simulink model "main_2022b"  (R2022b)
settings: Solver=ode4  StartTime=0.0  StopTime=0.1  FixedStep=deltat  RelTol=1e-3
model workspace (MAT data in the model file):
  Dutyfactor = Simulink.Parameter
  Dutyfactor.Value = 0.25
  Dutyfactor.DataType = 'double'
  Dutyfactor.Complexity = 'real'
  Dutyfactor.Dimensions = [1 1]
  LenghtOfBot = Simulink.Parameter
  LenghtOfBot.Value = 0.5
  LenghtOfBot.DataType = 'double'
  LenghtOfBot.Complexity = 'real'
  LenghtOfBot.Dimensions = [1 1]
  MomentOfInertia = Simulink.Parameter
  MomentOfInertia.Value = [0.41  0  0; 0  2.1  0; 0  0  2.1]
  MomentOfInertia.DataType = 'double'
  MomentOfInertia.Complexity = 'real'
  MomentOfInertia.Dimensions = [3 3]
  RelativePhase = Simulink.Parameter
  RelativePhase.Value = [0; 0.5; 0.75; 0.25]
  RelativePhase.DataType = 'double'
  RelativePhase.Complexity = 'real'
  RelativePhase.Dimensions = [4 1]
  WidthOfBot = Simulink.Parameter
  WidthOfBot.Value = 0.3
  WidthOfBot.DataType = 'double'
  WidthOfBot.Complexity = 'real'
  WidthOfBot.Dimensions = [1 1]
  cycleTime = Simulink.Parameter
  cycleTime.Value = 1
  cycleTime.DataType = 'double'
  cycleTime.Complexity = 'real'
  cycleTime.Dimensions = [1 1]
  deltat = Simulink.Parameter
  deltat.Value = 0.05
  deltat.DataType = 'double'
  deltat.Complexity = 'real'
  deltat.Dimensions = [1 1]
  gravity = Simulink.Parameter
  gravity.Value = [0; 0; -9.8]
  gravity.DataType = 'double'
  gravity.Complexity = 'real'
  gravity.Dimensions = [3 1]
  mass = Simulink.Parameter
  mass.Value = 45
  mass.DataType = 'double'
  mass.Complexity = 'real'
  mass.Dimensions = [1 1]
  nominal_height = Simulink.Parameter
  nominal_height.Value = 0.2
  nominal_height.DataType = 'double'
  nominal_height.Complexity = 'real'
  nominal_height.Dimensions = [1 1]
  number_of_timeStepsMPC = Simulink.Parameter
  number_of_timeStepsMPC.Value = 1
  number_of_timeStepsMPC.DataType = 'int8'
  number_of_timeStepsMPC.Complexity = 'real'
  number_of_timeStepsMPC.Dimensions = [1 1]
settings Model: Creator=user  LastModifiedBy=user
settings OptimizationCC: ReuseModelBlockBuffer=on

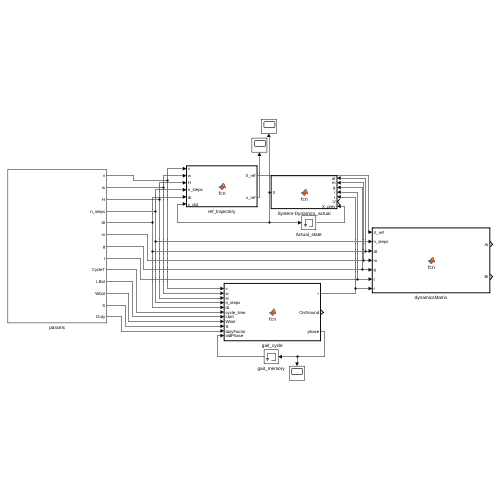
[thumbnail: Simulink's stored preview of the top-level diagram]
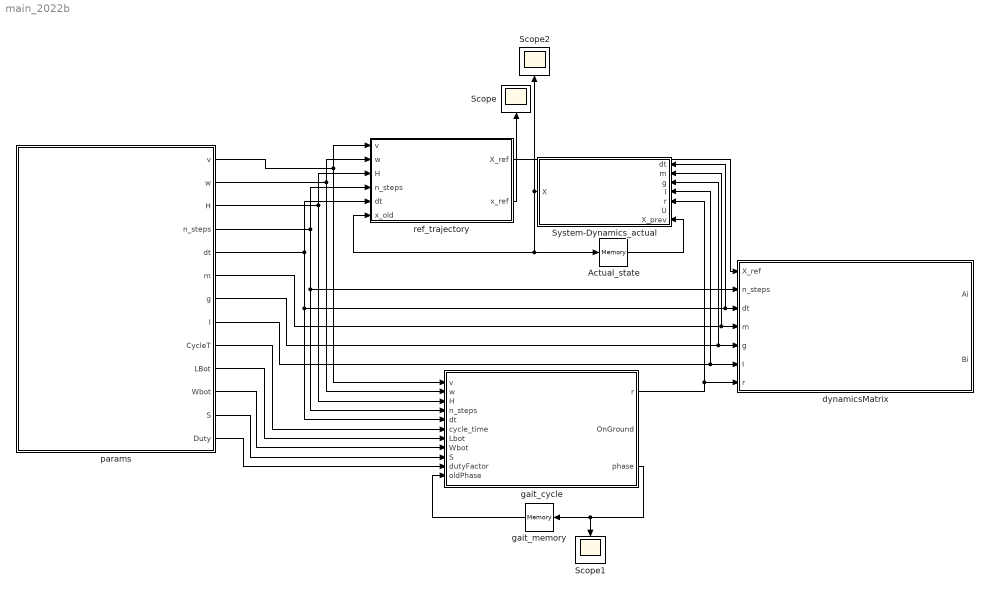
== system main_2022b ==
  Actual_state : Memory
  Scope : Scope
  Scope1 : Scope
  Scope2 : Scope
  System-Dynamics_actual : MATLAB Function  TreatAsAtomicUnit=on
  dynamicsMatrix : MATLAB Function  TreatAsAtomicUnit=on
  gait_cycle : MATLAB Function  TreatAsAtomicUnit=on
  gait_memory : Memory
  params : Subsystem
  ref_trajectory : MATLAB Function  TreatAsAtomicUnit=on
  wires:
  params/1(v) -> ref_trajectory/1(v), gait_cycle/1(v)
  params/2(w) -> gait_cycle/2(w), ref_trajectory/2(w)
  params/3(H) -> gait_cycle/3(H), ref_trajectory/3(H)
  params/4(n_steps) -> gait_cycle/4(n_steps), dynamicsMatrix/2(n_steps), ref_trajectory/4(n_steps)
  ref_trajectory/2(x_ref) -> Scope/1
  params/5(dt) -> gait_cycle/5(dt), dynamicsMatrix/3(dt), System-Dynamics_actual/1(dt), ref_trajectory/5(dt)
  params/9(CycleT) -> gait_cycle/6(cycle_time)
  params/10(LBot) -> gait_cycle/7(Lbot)
  params/11(Wbot) -> gait_cycle/8(Wbot)
  gait_memory/1 -> gait_cycle/11(oldPhase)
  ref_trajectory/1(X_ref) -> dynamicsMatrix/1(X_ref)
  params/6(m) -> dynamicsMatrix/4(m), System-Dynamics_actual/2(m)
  params/7(g) -> dynamicsMatrix/5(g), System-Dynamics_actual/3(g)
  gait_cycle/1(r) -> dynamicsMatrix/7(r), System-Dynamics_actual/5(r)
  params/12(S) -> gait_cycle/9(S)
  params/13(Duty) -> gait_cycle/10(dutyFactor)
  params/8(I) -> dynamicsMatrix/6(I), System-Dynamics_actual/4(I)
  System-Dynamics_actual/1(X) -> ref_trajectory/6(x_old), Actual_state/1, Scope2/1
  Actual_state/1 -> System-Dynamics_actual/7(X_prev)
  gait_cycle/3(phase) -> gait_memory/1, Scope1/1

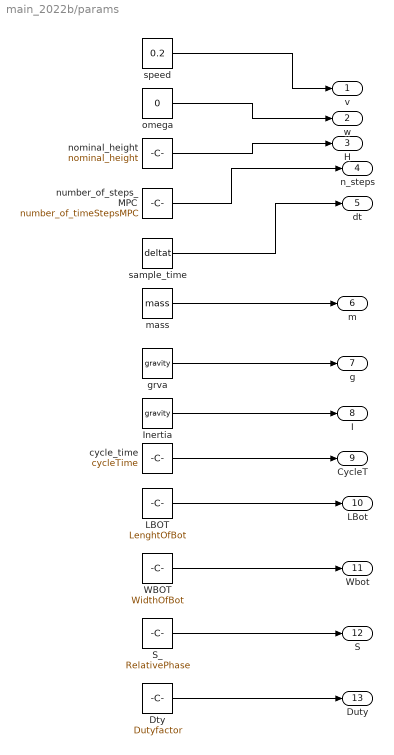
== system main_2022b/params ==
  Dty : Constant  Value=Dutyfactor
  Inertia : Constant  Value=gravity
  LBOT : Constant  Value=LenghtOfBot
  S_ : Constant  Value=RelativePhase
  WBOT : Constant  Value=WidthOfBot
  cycle_time : Constant  Value=cycleTime
  grva : Constant  Value=gravity
  mass : Constant  Value=mass
  nominal_height : Constant  Value=nominal_height
  number_of_steps_MPC : Constant  Value=number_of_timeStepsMPC
  omega : Constant  Value=0
  sample_time : Constant  Value=deltat
  speed : Constant  Value=0.2
  v : Outport
  w : Outport  Port=2
  H : Outport  Port=3
  n_steps : Outport  Port=4
  dt : Outport  Port=5
  m : Outport  Port=6
  g : Outport  Port=7
  I : Outport  Port=8
  CycleT : Outport  Port=9
  LBot : Outport  Port=10
  Wbot : Outport  Port=11
  S : Outport  Port=12
  Duty : Outport  Port=13
  wires:
  number_of_steps_MPC/1 -> n_steps/1
  omega/1 -> w/1
  nominal_height/1 -> H/1
  speed/1 -> v/1
  sample_time/1 -> dt/1
  cycle_time/1 -> CycleT/1
  LBOT/1 -> LBot/1
  WBOT/1 -> Wbot/1
  mass/1 -> m/1
  grva/1 -> g/1
  Dty/1 -> Duty/1
  S_/1 -> S/1
  Inertia/1 -> I/1

== matlab function main_2022b/gait_cycle ==
  data: v input; w input; H input; n_steps input; r output size=[3,4,500]; OnGround output size=[4,500]; dt input; cycle_time input; Lbot input; Wbot input; S input; dutyFactor input; oldPhase input; phase output double size=1
function [r,OnGround,phase] = fcn(v,w,H,n_steps,dt,cycle_time,Lbot,Wbot,S,dutyFactor,oldPhase)
    vr=(2*v+w*Wbot)/2;
    vl=(2*v-w*Wbot)/2;
    LstanceR=cycle_time*(1-dutyFactor)*vl;
    LstanceL=cycle_time*(1-dutyFactor)*vr;
    OnGround=zeros(4,n_steps);
    r=zeros(3,4,n_steps);
    phase=oldPhase;
    for k=1:n_steps
        phase=mod(phase+dt/cycle_time,1);
        for i=1:4           
            phase_leg=mod(phase+S(i),1);
            if(phase_leg>dutyFactor)
                OnGround(i,k)=1;
                if(i==1 || i==3)                 
                    r(:,i,k)=[LstanceL*(phase_leg/dutyFactor -0.5);0;0];             
                else
                    r(:,i,k)=[LstanceR*(phase_leg/dutyFactor -0.5);0;0];
                end                
            else
                r(:,i,k)=[0;0;H*0.25];
            end
        end
        r(:,:,k)=r(:,:,k)+[[Lbot/2;Wbot/2;-H],[Lbot/2;-Wbot/2;-H],[-Lbot/2;Wbot/2;-H],[-Lbot/2;-Wbot/2;-H]];
    end
    phase=mod(oldPhase+dt/cycle_time,1);
end

== matlab function main_2022b/ref_trajectory ==
  settings: updateMethod=DISCRETE  sampleTime=deltat
  data: v input; X_ref output double size=[12,500]; w input; H input; n_steps input; dt input; x_old input; x_ref output double size=12
function [X_ref,x_ref] = fcn(v,w,H,n_steps, dt,x_old)
    X_ref=zeros(12,n_steps);
    X_ref(:,1)=x_old;
    for i=0:(n_steps-1)
        X_ref(1,i+1)=X_ref(1,i+1)+v*dt*cos(X_ref(6,i+1));
        X_ref(2,i+1)=X_ref(2,i+1)+v*dt*sin(X_ref(6,i+1));
        X_ref(3,i+1)=H;        
        X_ref(7,i+1)=v*cos(X_ref(6,i+1));
        X_ref(8,i+1)=v*sin(X_ref(6,i+1));
        X_ref(6,i+1)=x_old(6)+w*dt;
        X_ref(12,i+1)=w;
        if(i<(n_steps-1))
            X_ref(:,i+2)=X_ref(:,i+1);
        end
    end
    x_ref=X_ref(:,1);
    % ground Air
    %Ri
end

== matlab function main_2022b/dynamicsMatrix ==
  data: X_ref input; n_steps input; dt input; Ai output double size=[12,12,500]; m input; g input; I input; r input; Bi output double size=[12,13,500]
function [Ai,Bi] = fcn(X_ref,n_steps,dt,m,g,I,r)
    Ai=zeros(12,12,n_steps);
    Bi=zeros(12,13,n_steps);
    I_=I^-1;
    for k=1:n_steps

        R=[cos(X_ref(6,k)), sin(X_ref(6,k)), 0;
          -sin(X_ref(6,k)), cos(X_ref(6,k)), 0;
                         0,               0, 1];

       A=[zeros(3), zeros(3),        R, zeros(3);
          zeros(3), zeros(3), zeros(3),  ones(3);
          zeros(3), zeros(3), zeros(3), zeros(3);
          zeros(3), zeros(3), zeros(3), zeros(3);];

       B=[       zeros(3),        zeros(3),        zeros(3),        zeros(3), zeros(3,1);
                 zeros(3),        zeros(3),        zeros(3),        zeros(3), zeros(3,1);
          I_*CP(r(:,1,k)), I_*CP(r(:,2,k)), I_*CP(r(:,3,k)), I_*CP(r(:,4,k)), zeros(3,1);
               ones(3)./m,      ones(3)./m,      ones(3)./m,      ones(3)./m,         g];
       
       Ai(:,:,k)=exp(A.*dt);
       Bi(:,:,k)=integral(@(t) exp(A.*t)*B,0,dt,"ArrayValued",true);

    end

    function R = CP(r)
        R=[0 -r(3) r(2);r(3) 0 -r(1);-r(2) r(1) 0];
    end
end

== matlab function main_2022b/System-Dynamics_actual ==
  data: dt input; X output; m input; g input; I input; r input; U input; X_prev input
function X  = fcn(dt,m,g,I,r,U,X_prev)     
    [t,y] = ode45(@dynamics_eq ,[0 dt],X_prev);
    X=y(end,:)';
    function dxdt=dynamics_eq(t,y)
        R=[cos(y(6)), sin(y(6)), 0;
         - sin(y(6)), cos(y(6)), 0;
                         0,               0, 1];
        I_=(R*I*R')^-1;        
        A=[zeros(3), zeros(3),        R, zeros(3);
           zeros(3), zeros(3), zeros(3),  ones(3);
           zeros(3), zeros(3), zeros(3), zeros(3);
           zeros(3), zeros(3), zeros(3), zeros(3);];
        
        B=[      zeros(3),        zeros(3),        zeros(3),        zeros(3), zeros(3,1);
                 zeros(3),        zeros(3),        zeros(3),        zeros(3), zeros(3,1);
          I_*CP(r(:,1,1)), I_*CP(r(:,2,1)), I_*CP(r(:,3,1)), I_*CP(r(:,4,1)), zeros(3,1);
               ones(3)./m,      ones(3)./m,      ones(3)./m,      ones(3)./m,         g];
        dxdt=A*y+B*U;
    end
end
